simulink model "project_detect"  (R2020b)
settings: Solver=FixedStepDiscrete  StartTime=0.0  StopTime=SimTime  RelTol=1e-3
values from neighbouring files (symbols this model uses):
  CorrFilter = transpose(CorrFilter)    [pulse_detect.m]
  RxSignal = RxSignal/scale1    [pulse_detect.m]
  threshold = 0.03    [pulse_detect.m]
  WindowLen = 11    [pulse_detect.m]
libraries: dspsrcs4 x2, dsphdlfiltering x1, simulink x1, hdlsllib x1
settings Model: DataTypeOverride=Off  Creator=cchung  LastModifiedBy=Aadhithan-PC
settings DataIOCC: SaveOutput=off  SaveTime=off
settings OptimizationCC: BlockReduction=off  ConditionallyExecuteInputs=off  DefaultParameterBehavior=Inlined
settings DebuggingCC: AlgebraicLoopMsg=error  SingleTaskRateTransMsg=error  PregeneratedLibrarySubsystemCodeDiagnostic=none  ArithmeticOperatorsInVariantConditions=warning
settings HardwareCC: ProdBitPerPointer=32  ProdBitPerSizeT=32  ProdBitPerPtrDiffT=32  ProdLargestAtomicFloat=None  ProdIntDivRoundTo=Undefined  ProdEndianess=Unspecified  ProdWordSize=32  ProdHWDeviceType=ASIC/FPGA->ASIC/FPGA  TargetBitPerPointer=64  TargetBitPerSizeT=64  TargetBitPerPtrDiffT=64  TargetLongLongMode=on  TargetIntDivRoundTo=Zero  TargetEndianess=LittleEndian  TargetWordSize=64  TargetHWDeviceType=Custom Processor->MATLAB Host Computer  ProdEqTarget=off
settings SFSimCC: SimUseLocalCustomCode=off  CustomCodeUndefinedFunction=UseInterfaceOnly
settings RTWCC: RTWUseLocalCustomCode=off

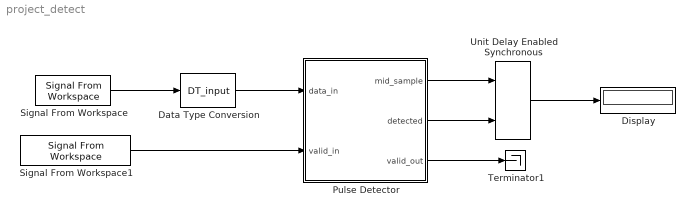
== system project_detect ==
  Data Type Conversion : DataTypeConversion  OutDataTypeStr=DT_input  RndMeth=Nearest  SaturateOnIntegerOverflow=on
  Display : Display
  Pulse Detector : Subsystem
  Signal From Workspace : dspsrcs4/Signal From Workspace  X=RxSignal  Ts=1  nsamps=1  OutputAfterFinalValue=Setting to zero  ignoreOrWarnInputAndFrameLengths=off  OutputFrames=off
  Signal From Workspace1 : dspsrcs4/Signal From Workspace  X=true(size(RxSignal))  Ts=1  nsamps=1  OutputAfterFinalValue=Setting to zero  ignoreOrWarnInputAndFrameLengths=off  OutputFrames=off
  Terminator1 : Terminator
  Unit Delay Enabled Synchronous : hdlsllib/Discrete/Unit Delay Enabled Synchronous  InitialCondition=0.0  SampleTime=-1
      settings: SourceProductBaseCode=SL
  wires:
  Unit Delay Enabled Synchronous/1 -> Display/1
  Signal From Workspace/1 -> Data Type Conversion/1
  Pulse Detector/1(mid_sample) -> Unit Delay Enabled Synchronous/1
  Pulse Detector/2(detected) -> Unit Delay Enabled Synchronous/2
  Signal From Workspace1/1 -> Pulse Detector/2(valid_in)
  Pulse Detector/3(valid_out) -> Terminator1/1
  Data Type Conversion/1 -> Pulse Detector/1(data_in)

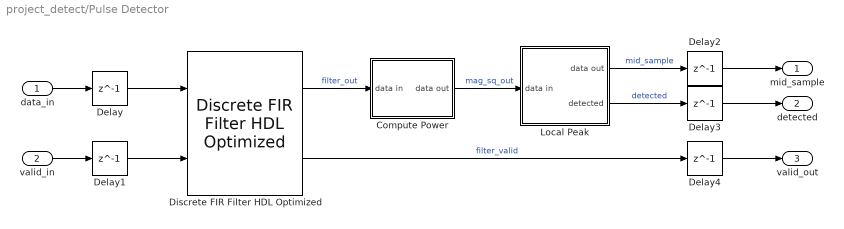
== system project_detect/Pulse Detector ==
  data_in : Inport
  valid_in : Inport  Port=2
  Compute Power : Subsystem
  Delay{,1..4} (5 alike) : Delay  DelayLength=1
  Discrete FIR Filter HDL Optimized : dsphdlfiltering/Discrete FIR Filter HDL Optimized  NumeratorSource=Property  Numerator=CorrFilter  NumeratorPrototype=[]  FilterStructure=Direct form systolic  SerializationOption=Minimum number of cycles between valid input samples  NumberOfCycles=2  NumberOfMultipliers=2  SimulateUsing=Code generation  roundingMode=Floor  overflowMode=off  CoefficientsDataTypeStr=DT_coeff  CoefficientsMin=[]  CoefficientsMax=[]  OutputMin=[]  OutputMax=[]  ResetInputPort=off  HDLGlobalReset=off
      settings: SourceProductBaseCode=DS
  Local Peak : Subsystem
  mid_sample : Outport
  detected : Outport  Port=2
  valid_out : Outport  Port=3
  wires:
  Local Peak/2(detected) -> Delay3/1  "detected"
  Discrete FIR Filter HDL Optimized/1 -> Compute Power/1(data in)  "filter_out"
  Compute Power/1(data out) -> Local Peak/1(data in)  "mag_sq_out"
  Local Peak/1(data out) -> Delay2/1  "mid_sample"
  data_in/1 -> Delay/1
  valid_in/1 -> Delay1/1
  Discrete FIR Filter HDL Optimized/2 -> Delay4/1  "filter_valid"
  Delay/1 -> Discrete FIR Filter HDL Optimized/1
  Delay1/1 -> Discrete FIR Filter HDL Optimized/2
  Delay2/1 -> mid_sample/1
  Delay3/1 -> detected/1
  Delay4/1 -> valid_out/1

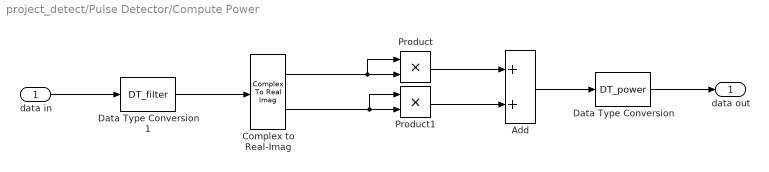
== system project_detect/Pulse Detector/Compute Power ==
  data in : Inport
  Add : Sum
  Complex to Real-Imag : ComplexToRealImag
  Data Type Conversion : DataTypeConversion  OutDataTypeStr=DT_power
  Data Type Conversion1 : DataTypeConversion  OutDataTypeStr=DT_filter
  Product : Product
  Product1 : Product
  data out : Outport  VectorParamsAs1DForOutWhenUnconnected=off
  wires:
  Complex to Real-Imag/1 -> Product/1, Product/2
  Complex to Real-Imag/2 -> Product1/1, Product1/2
  Product1/1 -> Add/2
  Product/1 -> Add/1
  Add/1 -> Data Type Conversion/1
  data in/1 -> Data Type Conversion1/1
  Data Type Conversion1/1 -> Complex to Real-Imag/1
  Data Type Conversion/1 -> data out/1

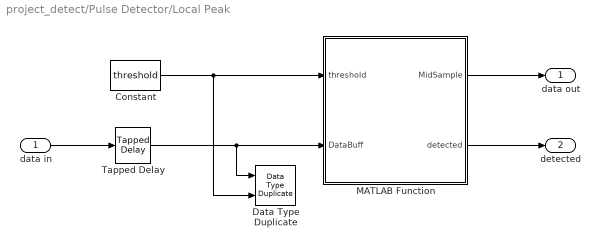
== system project_detect/Pulse Detector/Local Peak ==
  data in : Inport
  Constant : Constant  Value=threshold  OutDataTypeStr=Inherit: Inherit via back propagation  SampleTime=-1
  Data Type Duplicate : DataTypeDuplicate
  MATLAB Function : MATLAB Function  TreatAsAtomicUnit=on
  Tapped Delay : simulink/Discrete/Tapped Delay  vinit=0.0  samptime=-1  NumDelays=WindowLen  DelayOrder=Oldest  includeCurrent=off
  data out : Outport  VectorParamsAs1DForOutWhenUnconnected=off
  detected : Outport  Port=2  VectorParamsAs1DForOutWhenUnconnected=off
  wires:
  data in/1 -> Tapped Delay/1
  Tapped Delay/1 -> Data Type Duplicate/1, MATLAB Function/2(DataBuff)
  Constant/1 -> Data Type Duplicate/2, MATLAB Function/1(threshold)
  MATLAB Function/1(MidSample) -> data out/1
  MATLAB Function/2(detected) -> detected/1

== matlab function project_detect/Pulse Detector/Local Peak/MATLAB Function ==
  settings: fimath=fimath('RoundingMethod', 'Floor','OverflowAction', 'Wrap','ProductMode', 'FullPrecision', 'SumMode', 'FullPrecision')
  data: threshold input; DataBuff input; WindowLen parameter; MidSample output; detected output

% Hardware friendly implementation of peak finder
%
% Function inputs:
% * WindowLen - non-tunable parameter defined under Simulink->Edit Data
% * threhold  - input port (connected to constant)
% * DataBuff  - input port (buffering done using Simulink block)
%
% Function outputs:
% * "detected" is set when MidSample is local max

function [MidSample,detected] = fcn(threshold, DataBuff, WindowLen)
%#codegen


MidIdx = ceil(WindowLen/2);

% Compare each value in the window to the middle sample via subtraction
MidSample = DataBuff(MidIdx);
CompareOut = DataBuff - MidSample; % this is a vector

% if all values in the result are negative and the middle sample is
% greater than a threshold, it is a local max
if all(CompareOut <= 0) && (MidSample > threshold)
    detected = true;
else
    detected = false;
end
